simulink library "toSOMANET"  (R2016b)
settings: Solver=VariableStepAuto  StartTime=0.0  StopTime=10.0  RelTol=1e-3
libraries: LibraryModel x4
settings Model: Creator=Nathan  LastModifiedBy=Nathan

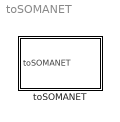
== system toSOMANET ==
  toSOMANET : Subsystem

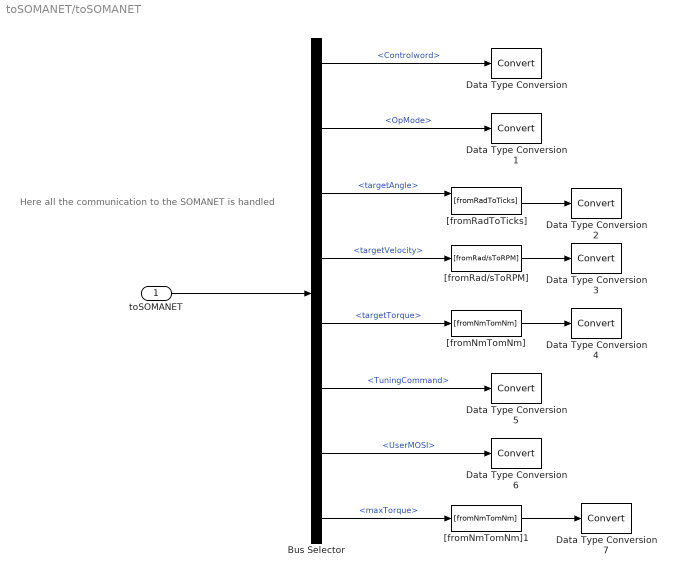
== system toSOMANET/toSOMANET ==
  note: Here all the communication to the SOMANET is handled
  toSOMANET : Inport  OutDataTypeStr=Bus: toSOMANET  BusOutputAsStruct=on
  Bus Selector : BusSelector  OutputSignals=Controlword,OpMode,targetAngle,targetVelocity,targetTorque,TuningCommand,UserMOSI,maxTorque
  Data Type Conversion{,1..7} (8 alike) : DataTypeConversion
  "[fromNmTomNm]" : LibraryModel/Conversions/[fromNmTomNm]
  "[fromNmTomNm]1" : LibraryModel/Conversions/[fromNmTomNm]
  "[fromRad/sToRPM]" : LibraryModel/Conversions/[fromRad//sToRPM]
  "[fromRadToTicks]" : LibraryModel/Conversions/[fromRadToTicks]
  wires:
  Bus Selector/5 -> "[fromNmTomNm]"/1  "<targetTorque>"
  Bus Selector/3 -> "[fromRadToTicks]"/1  "<targetAngle>"
  toSOMANET/1 -> Bus Selector/1
  Bus Selector/2 -> Data Type Conversion1/1  "<OpMode>"
  Bus Selector/6 -> Data Type Conversion5/1  "<TuningCommand>"
  "[fromNmTomNm]"/1 -> Data Type Conversion4/1
  "[fromNmTomNm]1"/1 -> Data Type Conversion7/1
  Bus Selector/4 -> "[fromRad/sToRPM]"/1  "<targetVelocity>"
  Bus Selector/8 -> "[fromNmTomNm]1"/1  "<maxTorque>"
  "[fromRadToTicks]"/1 -> Data Type Conversion2/1
  Bus Selector/7 -> Data Type Conversion6/1  "<UserMOSI>"
  "[fromRad/sToRPM]"/1 -> Data Type Conversion3/1
  Bus Selector/1 -> Data Type Conversion/1  "<Controlword>"
